simulink model "Smartinverter"  (R2024b)
settings: Solver=ode23t  StartTime=0.0  StopTime=1  MaxStep=1e-4  RelTol=1e-5
libraries: powerlib x9, powerlib_meascontrol x4, fuzblock x1, re_lib x1
settings Model: Creator=venka
settings SolverCC: ZeroCrossControl=DisableAll  ZeroCrossAlgorithm=Adaptive  AlgebraicLoopSolver=LineSearch
settings DataIOCC: SaveOutput=off  SignalLogging=off  DSMLogging=off  SaveTime=off  ReturnWorkspaceOutputs=off
settings DebuggingCC: MaxConsecutiveZCsMsg=none  UnconnectedInputMsg=warning  UnconnectedOutputMsg=warning  UnconnectedLineMsg=warning  ArithmeticOperatorsInVariantConditions=warning
settings ModelReferenceCC: EnableRefExpFcnMdlSchedulingChecks=on
settings SFSimCC: SimUseLocalCustomCode=off  CustomCodeUndefinedFunction=UseInterfaceOnly
settings RTWCC: RTWUseLocalCustomCode=off  GPUComputeCapability=3.5
settings CodeAppCC: StateflowObjectComments=on
settings ConfigComp: CovBoundaryAbsTol=1.0e-5
settings SimscapeCC: SimscapeNormalizeSystem=off

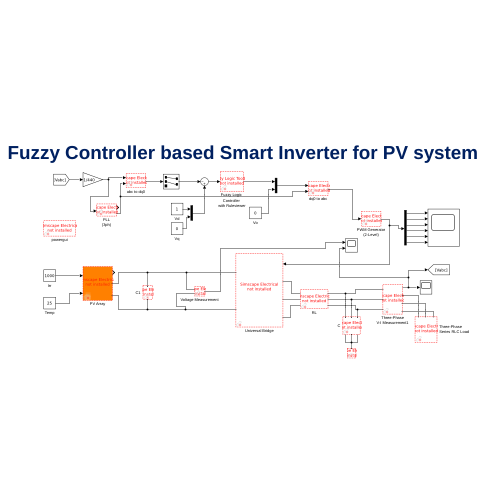
[thumbnail: Simulink's stored preview of the top-level diagram]
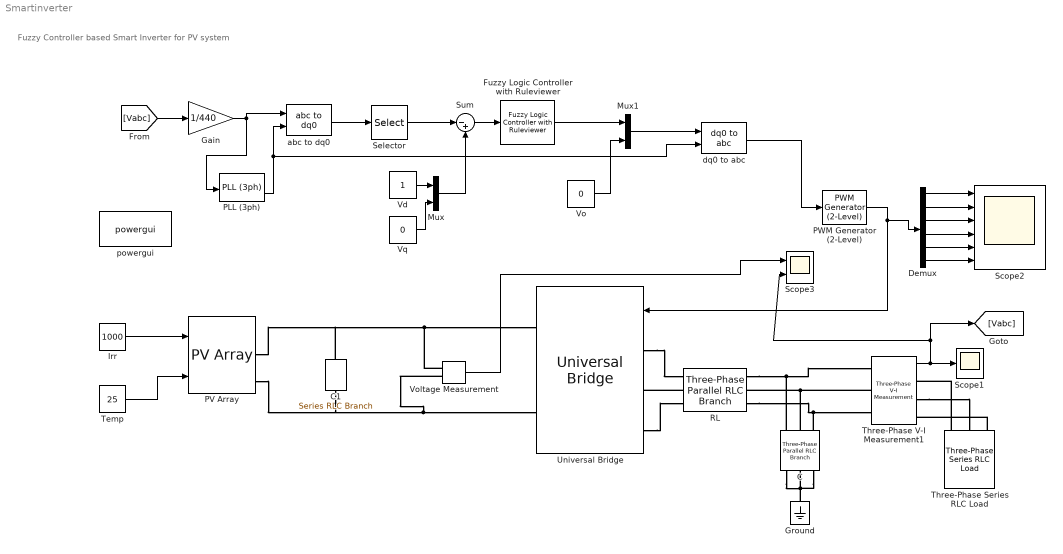
== system Smartinverter ==
  note: Fuzzy Controller based Smart Inverter for PV system
  C : powerlib/Elements/Three-Phase Parallel RLC Branch  LConnTagsString=A|B|C  RConnTagsString=A|B|C  BranchType=C  Resistance=1  Inductance=0.2e-2  Capacitance=550e-5  Measurements=None
      settings: SourceProductName=Simscape Power Systems
  C1 : powerlib/Elements/Series RLC Branch  LConnTagsString=__new0  RConnTagsString=__new0  BranchType=C  Resistance=1  Inductance=1e-3  SetiL0=off  InitialCurrent=0  Capacitance=470e-6  Setx0=off  InitialVoltage=0  Measurements=None
  Demux : Demux  Outputs=6
  Fuzzy Logic Controller with Ruleviewer : fuzblock/Fuzzy Logic  Controller  with Ruleviewer  fismatrix=SI  Ts=0.1
  Gain : Gain  Gain=1/440
  Ground : powerlib/Elements/Ground  LConnTagsString=a
  Irr : Constant  Value=1000
  Mux : Mux  Inputs=2
  Mux1 : Mux  Inputs=2
  PLL (3ph) : powerlib_meascontrol/PLL/PLL (3ph)  Fmin=45  Par_Init=[0, 50]  ParK=[180, 3200, 1]  TcD=1e-4  MaxRateChangeFreq=12  FilterCutOffFreq=25  Ts=0  AGC=on
  PV Array : re_lib/Solar/PV Array  Npar=40  Nser=10  PlotType=array @ 1000 W/m2 & specified temperatures  S_vec="[ 1000  500  100 ]"  Temp_C_vec="[ 45 25  ]"  ModuleName=1Soltech 1STH-215-P  PlotWhenSelected=off  Pm=213.15  Ncell=60  Voc=36.3  Isc=7.84  Vm=29  Im=7.35  beta_Voc_pc=-0.36099  alpha_Isc_pc=0.102  beta_Voc=-0.13104  alpha_Isc=0.007997  IL=7.8649  I0=2.9259e-10  nI=0.98117  Rsh=313.3991  Rs=0.39383  BAL=off  Tc=1e-6  Tfilter=5e-5
  PWM Generator (2-Level) : powerlib_meascontrol/Pulse & Signal Generators/PWM Generator (2-Level)  ModulatorType=Three-phase bridge (6 pulses)  ModulatorMode=Unsynchronized  Fc=27*50  Pc=90  nF=27  MinMax="[ -1  1 ]"  SamplingTechnique=Natural  ModulatingSignals=off  m=0.8  Freq=50  Phase=0  Ts=0  ShowCarrierOutport=off
      settings: SourceProductName=Simscape Power Systems
  RL : powerlib/Elements/Three-Phase Parallel RLC Branch  LConnTagsString=A|B|C  RConnTagsString=A|B|C  BranchType=RL  Resistance=1  Inductance=0.4e-2  Capacitance=1e-6  Measurements=None
      settings: SourceProductName=Simscape Power Systems
  Scope1 : Scope
  Scope2 : Scope  NumInputPorts=6
  Scope3 : Scope  NumInputPorts=2
  Selector : Selector  InputPortWidth=3  IndexOptions=Index vector (dialog)  Indices=[1 2]  OutputSizes=1
  Sum : Sum  Inputs=|-+
  Temp : Constant  Value=25
  Three-Phase Series RLC Load : powerlib/Elements/Three-Phase Series RLC Load  LConnTagsString=A|B|C  Configuration=Y (grounded)  NominalVoltage=440  Vabc=[1e3 1e3 1e3]  Vabcp=[1e3 1e3 1e3]  NominalFrequency=50  UnbalancedPower=off  ActivePower=500  InductivePower=100  CapacitivePower=0  Pabc=[10e3 9e3 11e3]  QLabc=[100 90 110]  QCabc=[100 90 110]  Pabcp=[10e3 9e3 11e3]  QLabcp=[100 90 110]  QCabcp=[100 90 110]  Measurements=None  LoadType=constant PQ
  Three-Phase V-I Measurement1 : powerlib/Measurements/Three-Phase V-I Measurement  VoltageMeasurement=phase-to-phase  SetLabelV=off  LabelV=Vabc  Vpu=off  VpuLL=off  CurrentMeasurement=no  SetLabelI=off  LabelI=Iabc  Ipu=off  Pbase=100e6  Vbase=500e3  OutputType=Complex  PhasorSimulation=off  PSBequivalent=0
  Universal Bridge : powerlib/Power Electronics/Universal Bridge  Arms=3  SnubberResistance=1e5  SnubberCapacitance=inf  Device=MOSFET / Diodes  Ron=1e-3  Lon=0  ForwardVoltages="[  0  0  ]"  ForwardVoltage=0  GTOparameters=[ 10e-6 , 20e-6 ]  IGBTparameters=[ 1e-6 , 2e-6 ]  Measurements=None  Measurements_2=None  converterType=Rectifier
  Vd : Constant
  Vo : Constant  Value=0
  Voltage Measurement : powerlib/Measurements/Voltage Measurement  PhasorSimulation=off  OutputType=Complex  PSBequivalent=0
  Vq : Constant  Value=0
  abc to dq0 : powerlib_meascontrol/Transformations/abc to dq0  Alignment=90 degrees behind phase A axis
  dq0 to abc : powerlib_meascontrol/Transformations/dq0 to abc  Alignment=90 degrees behind phase A axis
  powergui : powerlib/powergui  Priority=1  SimulationMode=Discrete  SampleTime=3e-7  frequency=60  Iterations=50  frequencyindice=0  Pbase=100e6  ErrMax=1e-4  UnitsV=kV  UnitsW=MW  buscounter=0  FunctionMessages=off  echomessages=off  EnableUseOfTLC=off  CurrentSourceSwitches=off  DisableSnubberDevices=off  DisableRonSwitches=off  DisableVfSwitches=off  DisplayEquations=off  SolverType=Tustin/Backward Euler (TBE)  Interpol=off  ExternalGateDelay=off  methode=off  Ts=100  x0status=blocks  SPID=on  SwTol=0  HookPort=off  RestoreLinks=warning  ResistiveCurrentMeasurement=off  Frange=[0:2:500]  Ylog=off  Xlog=on  ShowGrid=off  save=off  variable=ZData  structure=0  ZoomFFT=off  StartTime=0.0  cycles=1  DisplayStyle=1  fundamental=60  FreqAxis=off  MaxFrequency=1000  frequencyindicesteady=1  RmsSteady=1  display=off
  wires:
  Demux/6 -> Scope2/6
  Demux/5 -> Scope2/5
  Demux/4 -> Scope2/4
  Demux/3 -> Scope2/3
  Demux/1 -> Scope2/1
  Demux/2 -> Scope2/2
  PWM Generator (2-Level)/1 -> Demux/1, Universal Bridge/1
  Three-Phase V-I Measurement1/1 -> Scope3/2, [Vabc], Scope1/1
  [Vabc] -> Gain/1
  Gain/1 -> abc to dq0/1, PLL (3ph)/1
  abc to dq0/1 -> Selector/1
  Selector/1 -> Sum/1
  Vd/1 -> Mux/1
  Vq/1 -> Mux/2
  Mux/1 -> Sum/2
  Sum/1 -> Fuzzy Logic Controller with Ruleviewer/1
  Vo/1 -> Mux1/2
  Mux1/1 -> dq0 to abc/1
  PLL (3ph)/2 -> dq0 to abc/2, abc to dq0/2
  dq0 to abc/1 -> PWM Generator (2-Level)/1
  Voltage Measurement/1 -> Scope3/1
  Fuzzy Logic Controller with Ruleviewer/1 -> Mux1/1
  Irr/1 -> PV Array/1
  Temp/1 -> PV Array/2
  connections:
  Three-Phase V-I Measurement1/RConn2 -- Three-Phase Series RLC Load/LConn2
  Three-Phase Series RLC Load/LConn3 -- Three-Phase V-I Measurement1/RConn3
  Three-Phase Series RLC Load/LConn1 -- Three-Phase V-I Measurement1/RConn1
  Universal Bridge/LConn1 -- RL/LConn1
  RL/LConn2 -- Universal Bridge/LConn2
  Universal Bridge/LConn3 -- RL/LConn3
  RL/RConn1 -- C/LConn1 -- Three-Phase V-I Measurement1/LConn1
  Three-Phase V-I Measurement1/LConn2 -- C/LConn2 -- RL/RConn2
  RL/RConn3 -- C/LConn3 -- Three-Phase V-I Measurement1/LConn3
  Ground/LConn1 -- C/RConn3 -- C/RConn1 -- C/RConn2
  Voltage Measurement/LConn1 -- C1/LConn1 -- PV Array/RConn1 -- Universal Bridge/RConn1
  Voltage Measurement/LConn2 -- C1/RConn1 -- PV Array/RConn2 -- Universal Bridge/RConn2
